simulink model "robust_tracking_integral_dt"  (R2020b)
settings: Solver=ode45  StartTime=0.0  StopTime=5  FixedStep=T/10  RelTol=1e-3
undefined symbols (not defined in the file or in its folder): Beq_hat, ctrl, daq, DiscIntNeverNeededParam, drv, GAMMA, gbox, H0, J0, Jeq_hat, Ke, mot, N_u, N_x, PHI, rads2rpm, sens, step_size, T, tau_hat
settings Model: Creator=utente  LastModifiedBy=giuli
settings DataIOCC: ReturnWorkspaceOutputs=off

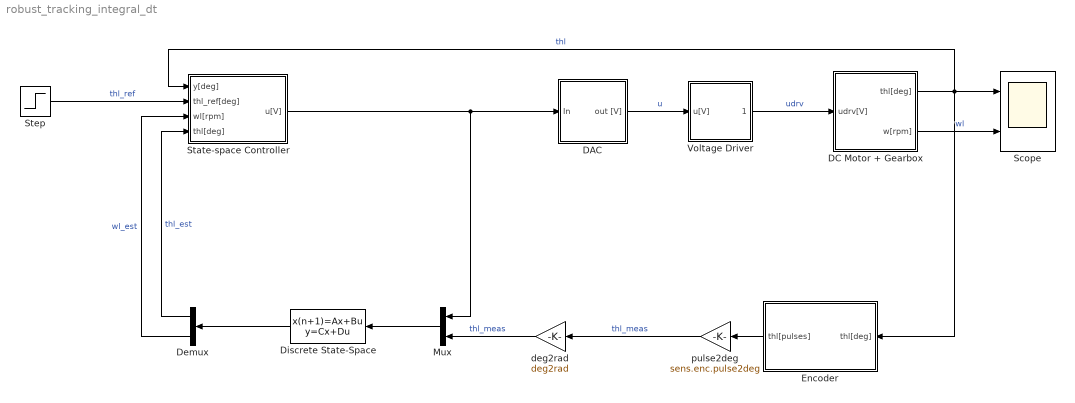
== system robust_tracking_integral_dt ==
  DAC : Subsystem
  DC Motor + Gearbox : Subsystem
  Demux : Demux  Outputs=2
  Discrete State-Space : DiscreteStateSpace  A=PHI  B=GAMMA  C=H0  D=J0  SampleTime=T
  Encoder : Subsystem
  Mux : Mux  Inputs=2
  Scope : Scope  NumInputPorts=2
  State-space Controller : Subsystem
  Step : Step  After=step_size  SampleTime=0
  Voltage Driver : Subsystem
  deg2rad : Gain  Gain=deg2rad
  pulse2deg : Gain  Gain=sens.enc.pulse2deg
  wires:
  DAC/1(out [V]) -> Voltage Driver/1(u[V])  "u"
  Voltage Driver/1(udrv[V]) -> DC Motor + Gearbox/1(udrv[V])  "udrv"
  Encoder/1(thl[pulses]) -> pulse2deg/1
  DC Motor + Gearbox/1(thl[deg]) -> State-space Controller/1(y[deg]), Scope/1, Encoder/1(thl[deg])  "thl"
  DC Motor + Gearbox/2(w[rpm]) -> Scope/2  "wl"
  Step/1 -> State-space Controller/2(thl_ref[deg])  "thl_ref"
  pulse2deg/1 -> deg2rad/1  "thl_meas"
  Mux/1 -> Discrete State-Space/1
  Demux/1 -> State-space Controller/4(thl[deg])  "thl_est"
  deg2rad/1 -> Mux/2  "thl_meas"
  Demux/2 -> State-space Controller/3(wl[rpm])  "wl_est"
  Discrete State-Space/1 -> Demux/1
  State-space Controller/1(u[V]) -> Mux/1, DAC/1(In)

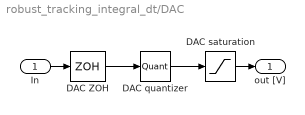
== system robust_tracking_integral_dt/DAC ==
  In : Inport
  DAC quantizer : Quantizer  QuantizationInterval=daq.dac.q
  DAC saturation : Saturate  UpperLimit=daq.dac.fs  LowerLimit=-daq.dac.fs
  DAC ZOH : ZeroOrderHold  SampleTime=0.001
  out [V] : Outport
  wires:
  DAC ZOH/1 -> DAC quantizer/1
  DAC quantizer/1 -> DAC saturation/1
  In/1 -> DAC ZOH/1
  DAC saturation/1 -> out [V]/1

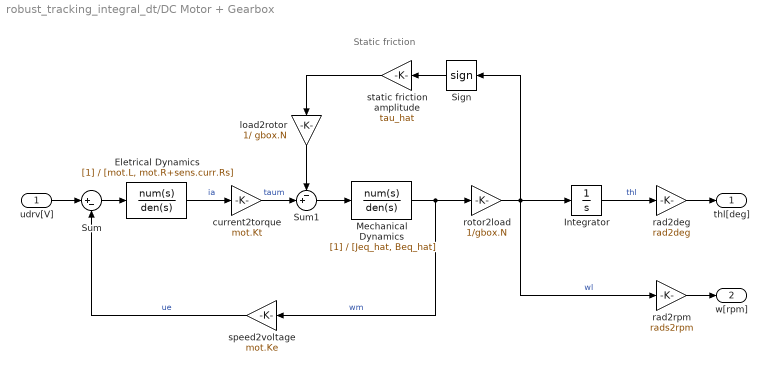
== system robust_tracking_integral_dt/DC Motor + Gearbox ==
  note: Static friction
  udrv[V] : Inport
  Eletrical Dynamics : TransferFcn  Denominator=[mot.L, mot.R+sens.curr.Rs]
  Integrator : Integrator
  Mechanical Dynamics : TransferFcn  Denominator=[Jeq_hat, Beq_hat]
  Sign : Signum  ZeroCross=off
  Sum : Sum  Inputs=|+-
  Sum1 : Sum  Inputs=-+|
  current2torque : Gain  Gain=mot.Kt
  load2rotor : Gain  Gain=1/ gbox.N
  rad2deg : Gain  Gain=rad2deg
  "rad2rpm " : Gain  Gain=rads2rpm
  rotor2load : Gain  Gain=1/gbox.N
  speed2voltage : Gain  Gain=mot.Ke
  static friction amplitude : Gain  Gain=tau_hat
  thl[deg] : Outport  VectorParamsAs1DForOutWhenUnconnected=off
  w[rpm] : Outport  Port=2  VectorParamsAs1DForOutWhenUnconnected=off
  wires:
  Eletrical Dynamics/1 -> current2torque/1  "ia"
  udrv[V]/1 -> Sum/1
  Sum/1 -> Eletrical Dynamics/1
  current2torque/1 -> Sum1/2  "taum"
  Sum1/1 -> Mechanical Dynamics/1
  Mechanical Dynamics/1 -> rotor2load/1, speed2voltage/1  "wm"
  rotor2load/1 -> Integrator/1, "rad2rpm "/1, Sign/1  "wl"
  Integrator/1 -> rad2deg/1  "thl"
  rad2deg/1 -> thl[deg]/1
  "rad2rpm "/1 -> w[rpm]/1
  static friction amplitude/1 -> load2rotor/1
  Sign/1 -> static friction amplitude/1
  speed2voltage/1 -> Sum/2  "ue"
  load2rotor/1 -> Sum1/1

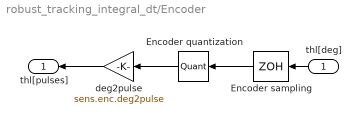
== system robust_tracking_integral_dt/Encoder ==
  thl[deg] : Inport
  Encoder quantization : Quantizer  QuantizationInterval=sens.enc.pulse2deg
  Encoder sampling : ZeroOrderHold  SampleTime=-1
  deg2pulse : Gain  Gain=sens.enc.deg2pulse
  thl[pulses] : Outport
  wires:
  thl[deg]/1 -> Encoder sampling/1
  Encoder quantization/1 -> deg2pulse/1
  Encoder sampling/1 -> Encoder quantization/1
  deg2pulse/1 -> thl[pulses]/1

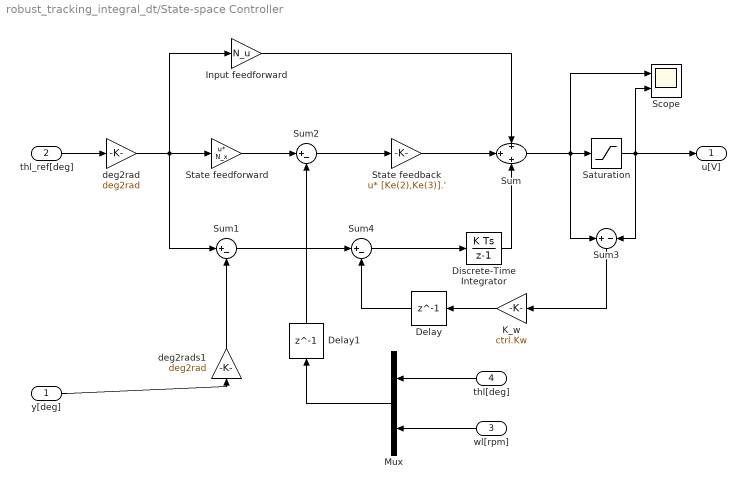
== system robust_tracking_integral_dt/State-space Controller ==
  y[deg] : Inport
  thl_ref[deg] : Inport  Port=2
  wl[rpm] : Inport  Port=3
  thl[deg] : Inport  Port=4
  Delay : Delay  DelayLength=1  InitialCondition=0
  Delay1 : Delay  DelayLength=1  InitialCondition=0
  Discrete-Time Integrator : DiscreteIntegrator  gainval=Ki  SampleTime=T  ICPrevOutput=DiscIntNeverNeededParam  ICPrevScaledInput=DiscIntNeverNeededParam
  Input feedforward : Gain  Gain=N_u
  K_w : Gain  Gain=ctrl.Kw
  Mux : Mux  Inputs=2
  Saturation : Saturate  UpperLimit=10  LowerLimit=-10
  Scope : Scope  NumInputPorts=2
  State feedback : Gain  Gain=[Ke(2),Ke(3)].'  Multiplication=Matrix(u*K)
  "State feedforward\t" : Gain  Gain=N_x  Multiplication=Matrix(u*K)
  Sum : Sum  Inputs=+|+|+
  Sum1 : Sum  Inputs=|+-
  Sum2 : Sum  Inputs=|+-
  Sum3 : Sum  Inputs=+|-
  Sum4 : Sum  Inputs=|+-
  deg2rad : Gain  Gain=deg2rad
  deg2rads1 : Gain  Gain=deg2rad
  u[V] : Outport
  wires:
  thl_ref[deg]/1 -> deg2rad/1
  deg2rad/1 -> Sum1/1, Input feedforward/1, "State feedforward\t"/1
  State feedback/1 -> Sum/2
  "State feedforward\t"/1 -> Sum2/1
  Sum2/1 -> State feedback/1
  Input feedforward/1 -> Sum/1
  thl[deg]/1 -> Mux/1
  wl[rpm]/1 -> Mux/2
  Mux/1 -> Delay1/1
  Discrete-Time Integrator/1 -> Sum/3
  Sum1/1 -> Sum4/1
  y[deg]/1 -> deg2rads1/1
  deg2rads1/1 -> Sum1/2
  Saturation/1 -> Sum3/2, Scope/2, u[V]/1
  Sum/1 -> Sum3/1, Scope/1, Saturation/1
  K_w/1 -> Delay/1
  Delay/1 -> Sum4/2
  Delay1/1 -> Sum2/2
  Sum4/1 -> Discrete-Time Integrator/1
  Sum3/1 -> K_w/1

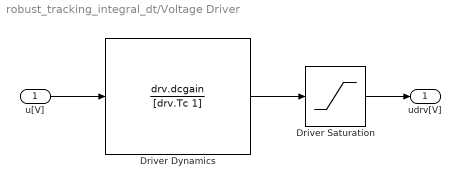
== system robust_tracking_integral_dt/Voltage Driver ==
  u[V] : Inport
  Driver Dynamics : TransferFcn  Numerator=drv.dcgain  Denominator=[drv.Tc 1]
  Driver Saturation : Saturate  UpperLimit=12  LowerLimit=-12
  udrv[V] : Outport
  wires:
  Driver Dynamics/1 -> Driver Saturation/1
  Driver Saturation/1 -> udrv[V]/1
  u[V]/1 -> Driver Dynamics/1
